simulink model "Assignment_01"  (R2023b)
settings: Solver=VariableStepAuto  StartTime=0.0  StopTime=17500  MaxStep=0.01  RelTol=1e-3
model workspace: external: MAT-File C:\Users\Frede\Documents\DTU\2024\Distributed Energy\Assignment 1\data_input_2024.mat (data not in the file)
undefined symbols (not defined in the file or in its folder): Ccell, Cth, NumCellsParallel, Rth, Tcell0
libraries: simulink x12
(part 2 of 2)

== system Assignment_01/Thermal dynamics2 ==
  note: here the thermal dynamic is assessed, taking as input Joule losses (RI^2)
      | and temperature difference between battery and outside (20 C)
  Joule losses (W) : Inport
  Tout (C) : Inport  Port=2
  1/Cth : Gain  Gain=1/Cth
  1/Rth : Gain  Gain=1/Rth
  Display29 : Display
  Display30 : Display
  Mux13 : Mux  Inputs=3
  Relay : Relay  OnSwitchValue=35  OffSwitchValue=25  OnOutputValue=4000
  Scope15 : Scope  NumInputPorts=2
  Sum15 : Sum  Inputs=|-+
  Sum16 : Sum  Inputs=|+--
  Tcell (C) : Integrator  InitialConditionSource=external  InitialCondition=Tcell0  ZeroCross=off
  Tbattery (C) : Outport  VectorParamsAs1DForOutWhenUnconnected=off
  wires:
  1/Rth/1 -> Sum16/2, Mux13/2  "Temp losses"
  Joule losses (W)/1 -> Sum16/1, Mux13/1  "Joule losses"
  Sum16/1 -> 1/Cth/1
  Sum15/1 -> 1/Rth/1
  1/Cth/1 -> Tcell (C)/1
  Mux13/1 -> Display29/1, Scope15/1
  Tcell (C)/1 -> Tbattery (C)/1, Scope15/2, Display30/1, Relay/1, Sum15/2
  Tout (C)/1 -> Tcell (C)/2, Sum15/1
  Relay/1 -> Mux13/3, Sum16/3  "cooling"
